simulink model "actuator_dynamics"  (R2019a)
settings: Solver=VariableStepAuto  StartTime=0.0  StopTime=1000  RelTol=1e-3
InitFcn:
  | initialize_lab_c
values from neighbouring files (symbols this model uses):
  A = [0, 	0	,  1.1320	, 	0		, -1.0000 ... (first row only)    [initialize_lab_c.m]    (also in initialize_lab_c_kalman.m; no_disturbances.mat = [0 0 0 0 0 0 -0.0538 0 0.0485 -0.2909 1.132 -0.1712 ... (25 )
  B = [	0		, 0		, 	0 ... (first row only)    [initialize_lab_c.m]    (also in initialize_lab_c_kalman.m; no_disturbances.mat = [0 -0.12 0 4.419 1.575 0 1 0 0 0 0 0 ... (15 elements, 5x3)])
  C = [  1, 0, 0, 0, 0 ... (first row only)    [initialize_lab_c.m]    (also in initialize_lab_c_kalman.m; no_disturbances.mat = [1 0 0 0 1 0 0 0 1 0 0 0 ... (15 elements, 3x5)])
  D = zeros(3)    [initialize_lab_c.m]    (also in initialize_lab_c_kalman.m; no_disturbances.mat = [0  0  0; 0  0  0; 0  0  0])
libraries: cstblocks x5
settings Model: Creator=marbla-6  LastModifiedBy=Martin

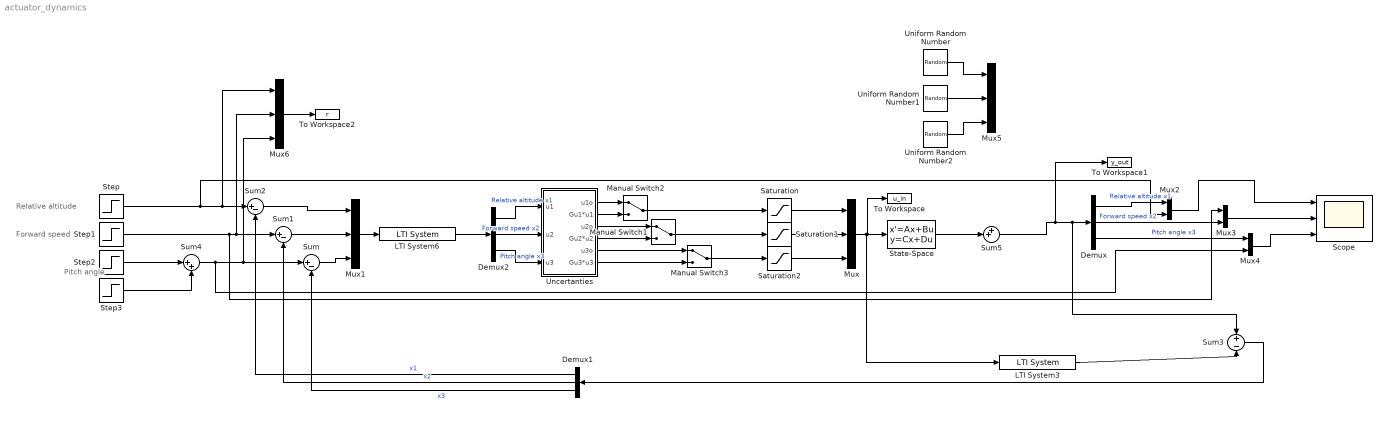
== system actuator_dynamics ==
  note: Pitch angle
  note: Forward speed
  note: Relative altitude
  Demux : Demux  Outputs=3
  Demux1 : Demux  Outputs=3
  Demux2 : Demux  Outputs=3
  LTI System3 : cstblocks/LTI System  sys=Gf  IC=[]
  LTI System6 : cstblocks/LTI System  sys=Q  IC=[]
  Manual Switch1 : ManualSwitch
  Manual Switch2 : ManualSwitch
  Manual Switch3 : ManualSwitch
  Mux{,1,5..6} (4 alike) : Mux  Inputs=3
  Mux2 : Mux  Inputs=2
  Mux3 : Mux  Inputs=2
  Mux4 : Mux  Inputs=2
  Saturation : Saturate  UpperLimit=900  LowerLimit=-900
  Saturation1 : Saturate  UpperLimit=15  LowerLimit=-15
  Saturation2 : Saturate  UpperLimit=90  LowerLimit=-90
  Scope : Scope  NumInputPorts=3
  State-Space : StateSpace  A=A  B=B  C=C  D=D  InitialCondition=0
  Step : Step  Time=10  After=25  SampleTime=0
  Step1 : Step  Time=500  After=2  SampleTime=0
  Step2 : Step  Time=700  After=-1  SampleTime=0
  Step3 : Step  Time=600  After=0  SampleTime=0
  Sum : Sum  Inputs=|+-
  Sum1 : Sum  Inputs=|+-
  Sum2 : Sum  Inputs=|+-
  Sum3 : Sum  Inputs=+-
  Sum4 : Sum  Inputs=|++
  Sum5 : Sum  Inputs=++|
  To Workspace : ToWorkspace  VariableName=u_in  SaveFormat=Timeseries  SampleTime=-1
  To Workspace1 : ToWorkspace  VariableName=y_out  SaveFormat=Timeseries  SampleTime=-1
  To Workspace2 : ToWorkspace  VariableName=r  SaveFormat=Timeseries  SampleTime=-1
  Uncertanties : Subsystem
  Uniform Random Number : UniformRandomNumber  SampleTime=0.1
  Uniform Random Number1 : UniformRandomNumber  Minimum=-.1  Maximum=.1  SampleTime=0.1
  Uniform Random Number2 : UniformRandomNumber  Minimum=-.1  Maximum=.1  SampleTime=0.1
  wires:
  Manual Switch3/1 -> Saturation2/1
  Manual Switch1/1 -> Saturation1/1
  Uncertanties/4(Gu2*u2) -> Manual Switch1/2
  Manual Switch2/1 -> Saturation/1
  Uncertanties/2(Gu1*u1) -> Manual Switch2/2
  Uncertanties/6(Gu3*u3) -> Manual Switch3/2
  Uncertanties/3(u2o) -> Manual Switch1/1
  Uncertanties/5(u3o) -> Manual Switch3/1
  Uncertanties/1(u1o) -> Manual Switch2/1
  Mux/1 -> LTI System3/1, State-Space/1, To Workspace/1
  Step/1 -> Mux2/2, Mux6/1, Sum2/1
  Step1/1 -> Mux3/2, Mux6/2, Sum1/1
  Demux1/1 -> Sum2/2  "x1"
  Demux1/2 -> Sum1/2  "x2"
  Demux1/3 -> Sum/2  "x3"
  Mux2/1 -> Scope/1
  Demux/1 -> Mux2/1  "Relative altitude x1"
  Demux/3 -> Mux4/1  "Pitch angle x3"
  Demux/2 -> Mux3/1  "Forward speed x2"
  Mux3/1 -> Scope/2
  Mux4/1 -> Scope/3
  Saturation1/1 -> Mux/2
  Saturation/1 -> Mux/1
  Saturation2/1 -> Mux/3
  Sum3/1 -> Demux1/1
  Sum4/1 -> Mux4/2, Mux6/3, Sum/1
  Step2/1 -> Sum4/1
  Step3/1 -> Sum4/2
  State-Space/1 -> Sum5/2
  LTI System3/1 -> Sum3/2
  Sum1/1 -> Mux1/2
  Sum2/1 -> Mux1/1
  Sum/1 -> Mux1/3
  Mux1/1 -> LTI System6/1
  Demux2/1 -> Uncertanties/1(u1)  "Relative altitude x1"
  Demux2/2 -> Uncertanties/2(u2)  "Forward speed x2"
  Demux2/3 -> Uncertanties/3(u3)  "Pitch angle x3"
  LTI System6/1 -> Demux2/1
  Sum5/1 -> Sum3/1, Demux/1, To Workspace1/1
  Uniform Random Number1/1 -> Mux5/2
  Uniform Random Number/1 -> Mux5/1
  Uniform Random Number2/1 -> Mux5/3
  Mux6/1 -> To Workspace2/1

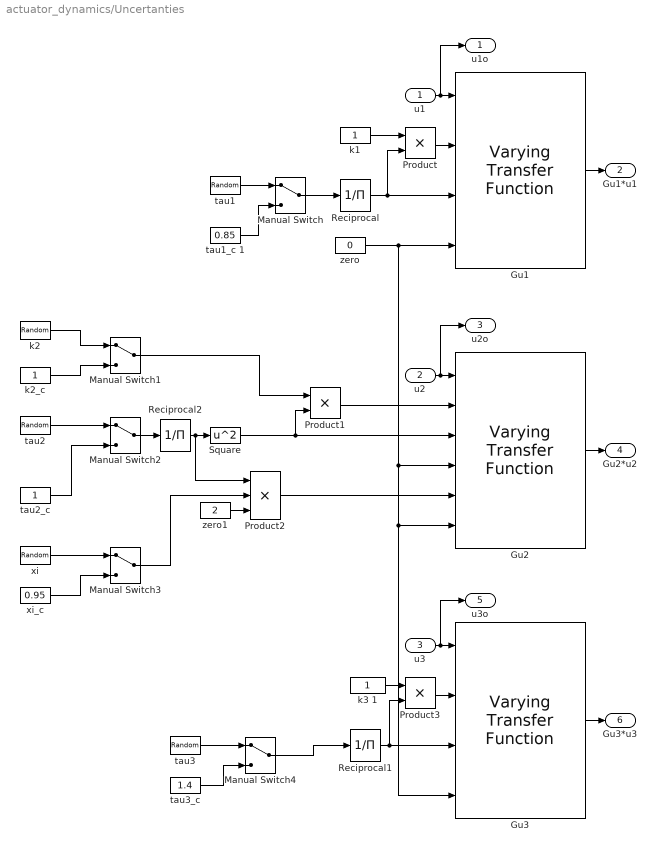
== system actuator_dynamics/Uncertanties ==
  u1 : Inport
  u2 : Inport  Port=2
  u3 : Inport  Port=3
  Gu1 : cstblocks/Linear Parameter Varying/Varying Transfer Function  N=1
      settings: SourceProductName=Control System Toolbox
  Gu2 : cstblocks/Linear Parameter Varying/Varying Transfer Function  N=2
      settings: SourceProductName=Control System Toolbox
  Gu3 : cstblocks/Linear Parameter Varying/Varying Transfer Function  N=1
      settings: SourceProductName=Control System Toolbox
  Manual Switch{,1..4} (5 alike) : ManualSwitch
  Product : Product
  Product1 : Product
  Product2 : Product  Inputs=3
  Product3 : Product
  Reciprocal : Product  Inputs=/
  Reciprocal1 : Product  Inputs=/
  Reciprocal2 : Product  Inputs=/
  Square : Math  Operator=square  SaturateOnIntegerOverflow=on
  "k1 " : Constant
  k2 : UniformRandomNumber  Minimum=0.9+1e-6  Maximum=1.1-1e-6  SampleTime=0.1
  k2_c : Constant
  k3 1 : Constant
  tau1 : UniformRandomNumber  Minimum=0.5+1e-6  Maximum=1.2-1e-6  SampleTime=0.1
  tau1_c 1 : Constant  Value=0.85
  tau2 : UniformRandomNumber  Minimum=0.5+1e-6  Maximum=2.5-1e-6  SampleTime=0.1
  tau2_c : Constant
  tau3 : UniformRandomNumber  Minimum=1+1e-6  Maximum=1.8-1e-6  SampleTime=0.1
  tau3_c : Constant  Value=1.4
  xi : UniformRandomNumber  Minimum=0.9+1e-6  Maximum=1-1e-6  SampleTime=0.1
  xi_c : Constant  Value=0.95
  zero : Constant  Value=0
  zero1 : Constant  Value=2
  u1o : Outport
  Gu1*u1 : Outport  Port=2
  u2o : Outport  Port=3
  Gu2*u2 : Outport  Port=4
  u3o : Outport  Port=5
  Gu3*u3 : Outport  Port=6
  wires:
  Gu2/1 -> Gu2*u2/1
  Manual Switch3/1 -> Product2/2
  tau3_c/1 -> Manual Switch4/2
  u1/1 -> u1o/1, Gu1/1
  Reciprocal/1 -> Gu1/3, Product/2
  Gu3/1 -> Gu3*u3/1
  Reciprocal1/1 -> Gu3/3, Product3/2
  Product1/1 -> Gu2/2
  Square/1 -> Gu2/3, Product1/2
  k2/1 -> Manual Switch1/1
  k3 1/1 -> Product3/1
  xi_c/1 -> Manual Switch3/2
  zero1/1 -> Product2/3
  Manual Switch/1 -> Reciprocal/1
  Manual Switch4/1 -> Reciprocal1/1
  Reciprocal2/1 -> Product2/1, Square/1
  xi/1 -> Manual Switch3/1
  zero/1 -> Gu1/4, Gu3/4, Gu2/6, Gu2/4
  tau2_c/1 -> Manual Switch2/2
  Product3/1 -> Gu3/2
  "k1 "/1 -> Product/1
  Manual Switch2/1 -> Reciprocal2/1
  u2/1 -> u2o/1, Gu2/1
  Product/1 -> Gu1/2
  Product2/1 -> Gu2/5
  k2_c/1 -> Manual Switch1/2
  tau1/1 -> Manual Switch/1
  Manual Switch1/1 -> Product1/1
  tau3/1 -> Manual Switch4/1
  u3/1 -> u3o/1, Gu3/1
  tau1_c 1/1 -> Manual Switch/2
  tau2/1 -> Manual Switch2/1
  Gu1/1 -> Gu1*u1/1
